simulink model "mass_spring"  (R2024a)
settings: Solver=FixedStepAuto  StartTime=0.0  StopTime=50  FixedStep=0.01  RelTol=1e-3
settings Model: Creator=gladstonjoseph  LastModifiedBy=gladstonjoseph

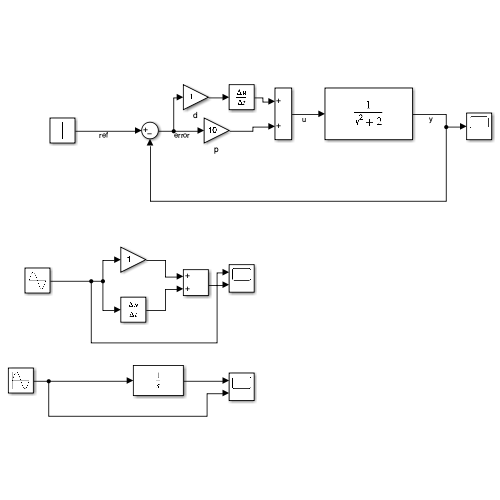
[thumbnail: Simulink's stored preview of the top-level diagram]
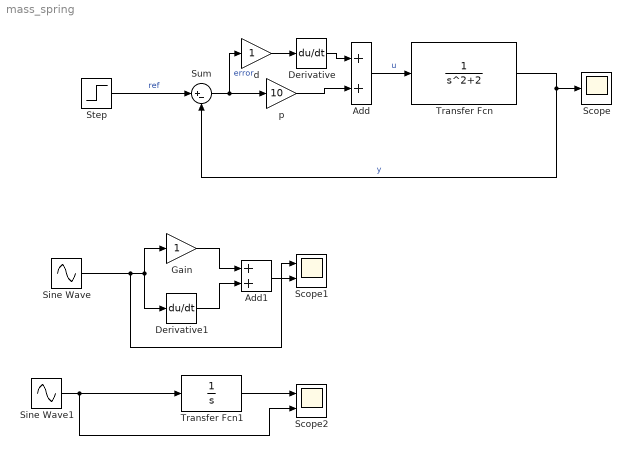
== system mass_spring ==
  Add : Sum
  Add1 : Sum
  Derivative : Derivative
  Derivative1 : Derivative
  Gain : Gain
  Scope : Scope
  Scope1 : Scope  NumInputPorts=2
  Scope2 : Scope  NumInputPorts=2
  Sine Wave : Sin  SampleTime=0
  Sine Wave1 : Sin  SampleTime=0
  Step : Step  SampleTime=0
  Sum : Sum  Inputs=|+-
  Transfer Fcn : TransferFcn  Denominator=[1 0 2]
  Transfer Fcn1 : TransferFcn  Denominator=[1 0]
  d : Gain
  p : Gain  Gain=10
  wires:
  Transfer Fcn/1 -> Sum/2, Scope/1  "y"
  Sum/1 -> d/1, p/1  "error"
  Step/1 -> Sum/1  "ref"
  p/1 -> Add/2
  d/1 -> Derivative/1
  Derivative/1 -> Add/1
  Add/1 -> Transfer Fcn/1  "u"
  Gain/1 -> Add1/1
  Derivative1/1 -> Add1/2
  Add1/1 -> Scope1/1
  Sine Wave/1 -> Scope1/2, Derivative1/1, Gain/1
  Transfer Fcn1/1 -> Scope2/1
  Sine Wave1/1 -> Scope2/2, Transfer Fcn1/1
